simulink model "Fullcar_model_outdated"  (R2018b)
settings: Solver=FixedStepAuto  StartTime=0.0  StopTime=inf  FixedStep=0.002  RelTol=1e-3
PreLoadFcn:
  | fullcar_data
values from neighbouring files (symbols this model uses):
  Body_m = 1106.284    [fullcar_data.m]
  C_max = 4000    [fullcar_data.m]
  C_min = 300    [fullcar_data.m]
  N = L/B    [Fcn_General_Road.m]    (also in Road_Generator_Fullcar_final.m = floor(length(z_Rough_LH)/20); autoSaver.m = length(Road_z))
  s = (cnt - 1)*N    [Road_Generator_Fullcar_final.m]
  sat_limit = 1000    [fullcar_data.m]    (also in skyhook.m = 500)
  TW = 1568*0.001    (= 1.568)    [fullcar_data.m]
  WB = 2650*0.001    (= 2.65)    [fullcar_data.m]
  Whl_m_Frt = 101.488/2    (= 50.744)    [fullcar_data.m]
  Whl_m_Rr = 86.718/2    (= 43.359)    [fullcar_data.m]
  Y = zeros(N,4)    [autoSaver.m]
undefined symbols (not defined in the file or in its folder): X, Z
libraries: nesl_utility x43, sm_lib x36, sharedtransform x1
(part 2 of 2)

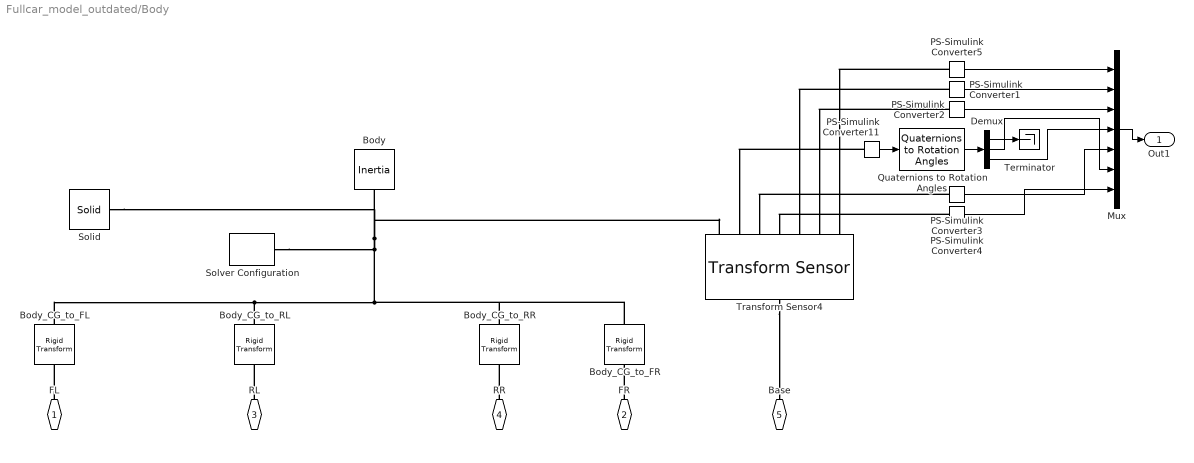
== system Fullcar_model_outdated/Body ==
  Body : sm_lib/Body Elements/Inertia  InertiaType=Custom  Mass=Body_m  MassUnits=kg  CenterOfMass=[0 0 0]  CenterOfMassUnits=m  MomentsOfInertia=[1 1 1]  MomentsOfInertiaUnits=kg*m^2  ProductsOfInertia=[0 0 0]  ProductsOfInertiaUnits=kg*m^2  GraphicType=Marker  MarkerShape=Inertia  MarkerSize=20  GraphicVisPropType=SimpleVisualProperties  GraphicDiffuseColor=[0.5 0.5 0.5]  GraphicSpecularColor=[0.5 0.5 0.5 1.0]  GraphicAmbientColor=[0.15 0.15 0.15 1.0]  GraphicEmissiveColor=[0.0 0.0 0.0 1.0]  GraphicShininess=75  GraphicOpacity=1.0
  Body_CG_to_FL : sm_lib/Frames and Transforms/Rigid Transform  TranslationMethod=Cartesian  TranslationStandardOffset=0  TranslationLengthUnit=m  TranslationStandardAxis=+Z  TranslationCartesianOffset=Body_CG_to_FL  TranslationROffset=0  TranslationROffsetUnits=m  TranslationZOffset=0  TranslationZOffsetUnits=m  TranslationThetaOffset=0  TranslationThetaOffsetUnits=deg  RotationMethod=None  RotationAngleUnits=deg  RotationStandardAxis=+Z  RotationAngle=0.0  RotationArbitraryAxis=[0 0 1]  FollAlignAxisA=+X  BaseAlignAxisA=+Y  FollAlignAxisB=+Y  BaseAlignAxisB=+Z  RotationSequenceAxes=FollowerAxes  RotationSequence=XYX  RotationSequenceAngles=[0 0 0]  RotationSequenceAnglesUnits=deg  RotationMatrix=[1 0 0; 0 1 0; 0 0 1]
  Body_CG_to_FR : sm_lib/Frames and Transforms/Rigid Transform  TranslationMethod=Cartesian  TranslationStandardOffset=0  TranslationLengthUnit=m  TranslationStandardAxis=+Z  TranslationCartesianOffset=Body_CG_to_FR  TranslationROffset=0  TranslationROffsetUnits=m  TranslationZOffset=0  TranslationZOffsetUnits=m  TranslationThetaOffset=0  TranslationThetaOffsetUnits=deg  RotationMethod=None  RotationAngleUnits=deg  RotationStandardAxis=+Z  RotationAngle=0.0  RotationArbitraryAxis=[0 0 1]  FollAlignAxisA=+X  BaseAlignAxisA=+Y  FollAlignAxisB=+Y  BaseAlignAxisB=+Z  RotationSequenceAxes=FollowerAxes  RotationSequence=XYX  RotationSequenceAngles=[0 0 0]  RotationSequenceAnglesUnits=deg  RotationMatrix=[1 0 0; 0 1 0; 0 0 1]
  Body_CG_to_RL : sm_lib/Frames and Transforms/Rigid Transform  TranslationMethod=Cartesian  TranslationStandardOffset=0  TranslationLengthUnit=m  TranslationStandardAxis=+Z  TranslationCartesianOffset=Body_CG_to_RL  TranslationROffset=0  TranslationROffsetUnits=m  TranslationZOffset=0  TranslationZOffsetUnits=m  TranslationThetaOffset=0  TranslationThetaOffsetUnits=deg  RotationMethod=None  RotationAngleUnits=deg  RotationStandardAxis=+Z  RotationAngle=0.0  RotationArbitraryAxis=[0 0 1]  FollAlignAxisA=+X  BaseAlignAxisA=+Y  FollAlignAxisB=+Y  BaseAlignAxisB=+Z  RotationSequenceAxes=FollowerAxes  RotationSequence=XYX  RotationSequenceAngles=[0 0 0]  RotationSequenceAnglesUnits=deg  RotationMatrix=[1 0 0; 0 1 0; 0 0 1]
  Body_CG_to_RR : sm_lib/Frames and Transforms/Rigid Transform  TranslationMethod=Cartesian  TranslationStandardOffset=0  TranslationLengthUnit=m  TranslationStandardAxis=+Z  TranslationCartesianOffset=Body_CG_to_RR  TranslationROffset=0  TranslationROffsetUnits=m  TranslationZOffset=0  TranslationZOffsetUnits=m  TranslationThetaOffset=0  TranslationThetaOffsetUnits=deg  RotationMethod=None  RotationAngleUnits=deg  RotationStandardAxis=+Z  RotationAngle=0.0  RotationArbitraryAxis=[0 0 1]  FollAlignAxisA=+X  BaseAlignAxisA=+Y  FollAlignAxisB=+Y  BaseAlignAxisB=+Z  RotationSequenceAxes=FollowerAxes  RotationSequence=XYX  RotationSequenceAngles=[0 0 0]  RotationSequenceAnglesUnits=deg  RotationMatrix=[1 0 0; 0 1 0; 0 0 1]
  Demux : Demux  Outputs=3
  Mux : Mux  Inputs=7
  PS-Simulink Converter{1..5,11} (6 alike) : nesl_utility/PS-Simulink Converter  PhysicalDomain=network_engine_domain  SubClassName=ps_output  LeftPortType=input  RightPortType=output  PseudoPeriodic=off  Frequencies=[]  Unit=1  AffineConversion=off
  Quaternions to Rotation Angles : sharedtransform/Quaternions to Rotation Angles  rotationOrder=ZYX  aMode=aMode
      settings: SourceProductBaseCode=AE
  Solid : sm_lib/Body Elements/Solid  InertiaType=CalculateFromGeometry  Mass=1  MassUnits=kg  CenterOfMass=[0 0 0]  CenterOfMassUnits=m  MomentsOfInertia=[1 1 1]  MomentsOfInertiaUnits=kg*m^2  ProductsOfInertia=[0 0 0]  ProductsOfInertiaUnits=kg*m^2  BasedOnType=Density  Density=1000  DensityUnits=kg/m^3  DoExposeReferenceFrame=on  SerializedFrames=<Frames/>  GraphicType=FromGeometry  MarkerShape=Sphere  MarkerSize=10  GraphicVisPropType=SimpleVisualProperties  GraphicDiffuseColor=[0.8 1.0 0.8]  GraphicSpecularColor=[0.5 0.5 0.5 1.0]  GraphicAmbientColor=[0.15 0.15 0.15 1.0]  GraphicEmissiveColor=[0.0 0.0 0.0 1.0]  GraphicShininess=75  GraphicOpacity=0.5  GeometryShape=Brick  RectangleSize=[1 1]  RectangleSizeUnits=m  BrickDimensions=[WB TW 0.5]  BrickDimensionUnits=m  CylinderRadius=1  CylinderRadiusUnits=m  CylinderLength=1  CylinderLengthUnits=m  SphereRadius=1  SphereRadiusUnits=m  EllipsoidRadii=[1 1 1]  EllipsoidRadiiUnits=m  ExtrusionCrossSection=[1 1; -1 1; -1 -1; 1 -1]  ExtrusionCrossSectionUnits=m  ExtrusionLength=1  ExtrusionLengthUnits=m  PolygonNumSides=3  PolygonOuterRadius=1  PolygonOuterRadiusUnits=m  ExtGeomFileType=STEP  ExtGeomFileUnits=m  RevolutionCrossSection=[1 1; 1 -1; 2 -1; 2 1]  RevolutionCrossSectionUnits=m  RevolutionExtent=Full  RevolutionAngle=180  RevolutionAngleUnits=deg
  Solver Configuration : nesl_utility/Solver Configuration  PhysicalDomain=network_engine_domain  SubClassName=solver  LeftPortType=input  RightPortType=generic  Tones=[]  Harmonics=[]  SimulateNoise=off  Profile=off  UseLocalSampling=off  EnableSwitchedLinearOptims=on  FrequencyDomain=off  UseCCode=off  RelTol=0.001  AbsTol=1e-06  MinStep=1e-09  ToWorkspace=off  RevertToSquareIcSolve=off  NumHomotopyIterations=100  PhasorMode=off  PhasorModeNumHarmonics=1  DoDC=off  ResidualTolerance=1e-09  UseLocalSolver=off  LocalSolverChoice=NE_BACKWARD_EULER_ADVANCER  LocalSolverSampleTime=0.001  DoFixedCost=off  MaxNonlinIter=3  MaxModeIter=2  LinearAlgebra=auto  EquationFormulation=NE_TIME_EF  DelaysMemoryBudget=1024  AutomaticFiltering=on  FilteringTimeConstant=0.001  PartitionStorageMethod=AS_NEEDED  PartitionMemoryBudget=1024  PartitionMethod=FAST
  Terminator : Terminator
  Transform Sensor4 : sm_lib/Frames and Transforms/Transform Sensor  MeasurementFrame=World  SenseAngle=off  SenseAxis=off  SenseAngle1=off  SenseAngle2=off  SenseAngle3=off  SenseQ=on  SenseR=off  SenseOmegaX=on  SenseOmegaY=on  SenseOmegaZ=off  SenseOmega1=off  SenseOmega2=off  SenseOmega3=off  SenseQDot=off  SenseRDot=off  SenseAlphaX=off  SenseAlphaY=off  SenseAlphaZ=off  SenseAlpha1=off  SenseAlpha2=off  SenseAlpha3=off  SenseQDDot=off  SenseRDDot=off  SenseX=off  SenseY=off  SenseZ=on  SenseRad=off  SenseAzim=off  SenseDist=off  SenseInc=off  SenseXDot=off  SenseYDot=off  SenseZDot=on  SenseRadDot=off  SenseAzimDot=off  SenseDistDot=off  SenseIncDot=off  SenseXDDot=off  SenseYDDot=off  SenseZDDot=on  SenseRadDDot=off  SenseAzimDDot=off  SenseDistDDot=off  SenseIncDDot=off
  FL : PMIOPort  Side=Left
  FR : PMIOPort  Port=2  Side=Right
  RL : PMIOPort  Port=3  Side=Left
  RR : PMIOPort  Port=4  Side=Right
  Base : PMIOPort  Port=5  Side=Right
  Out1 : Outport
  wires:
  Demux/3 -> Mux/4
  PS-Simulink Converter11/1 -> Quaternions to Rotation Angles/1
  Quaternions to Rotation Angles/1 -> Demux/1
  Demux/1 -> Terminator/1
  PS-Simulink Converter2/1 -> Mux/3
  PS-Simulink Converter3/1 -> Mux/5
  Mux/1 -> Out1/1
  Demux/2 -> Mux/6
  PS-Simulink Converter1/1 -> Mux/2
  PS-Simulink Converter4/1 -> Mux/7
  PS-Simulink Converter5/1 -> Mux/1
  connections:
  Body_CG_to_FL/LConn1 -- Body_CG_to_RL/LConn1 -- Body_CG_to_RR/LConn1 -- Body_CG_to_FR/LConn1 -- Body/RConn1 -- Solid/RConn1 -- Transform Sensor4/RConn1 -- Solver Configuration/RConn1
  FR/RConn1 -- Body_CG_to_FR/RConn1
  FL/RConn1 -- Body_CG_to_FL/RConn1
  RL/RConn1 -- Body_CG_to_RL/RConn1
  RR/RConn1 -- Body_CG_to_RR/RConn1
  PS-Simulink Converter1/LConn1 -- Transform Sensor4/RConn5
  PS-Simulink Converter3/LConn1 -- Transform Sensor4/RConn3
  PS-Simulink Converter4/LConn1 -- Transform Sensor4/RConn4
  PS-Simulink Converter2/LConn1 -- Transform Sensor4/RConn6
  PS-Simulink Converter11/LConn1 -- Transform Sensor4/RConn2
  Transform Sensor4/LConn1 -- Base/RConn1
  PS-Simulink Converter5/LConn1 -- Transform Sensor4/RConn7

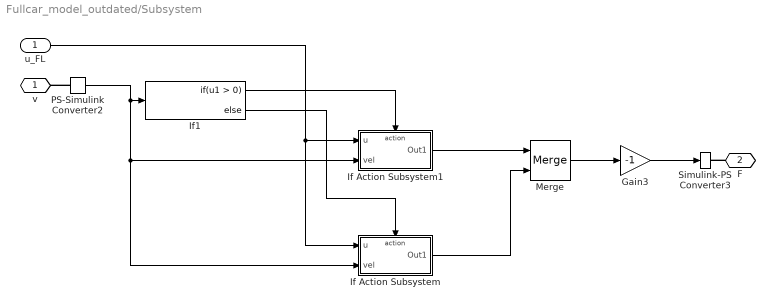
== system Fullcar_model_outdated/Subsystem ==
  "u_FL " : Inport
  Gain3 : Gain  Gain=-1
  If Action Subsystem : Subsystem  TreatAsAtomicUnit=on
  If Action Subsystem1 : Subsystem  TreatAsAtomicUnit=on
  If1 : If
  Merge : Merge
  PS-Simulink Converter2 : nesl_utility/PS-Simulink Converter  PhysicalDomain=network_engine_domain  SubClassName=ps_output  LeftPortType=input  RightPortType=output  PseudoPeriodic=off  Frequencies=[]  Unit=1  AffineConversion=off
  Simulink-PS Converter3 : nesl_utility/Simulink-PS Converter  PhysicalDomain=network_engine_domain  SubClassName=ps_input  LeftPortType=input  RightPortType=output  PseudoPeriodic=off  Frequencies=[]  NoiseDistribution=none  NoiseParameters=[]  Unit=1  AffineConversion=off  FilteringAndDerivatives=provide  SimscapeFilterOrder=1  InputFilterTimeConstant=0.001  UdotUserProvided=0
  "v " : PMIOPort  Side=Left
  F : PMIOPort  Port=2  Side=Right
  wires:
  PS-Simulink Converter2/1 -> If Action Subsystem/2("vel "), If Action Subsystem1/2("vel "), If1/1
  If1/1 -> If Action Subsystem1/Action
  Merge/1 -> Gain3/1
  If Action Subsystem1/1(Out1) -> Merge/1
  If1/2 -> If Action Subsystem/Action
  "u_FL "/1 -> If Action Subsystem/1("u "), If Action Subsystem1/1("u ")
  If Action Subsystem/1(Out1) -> Merge/2
  Gain3/1 -> Simulink-PS Converter3/1
  connections:
  PS-Simulink Converter2/LConn1 -- "v "/RConn1
  F/RConn1 -- Simulink-PS Converter3/RConn1

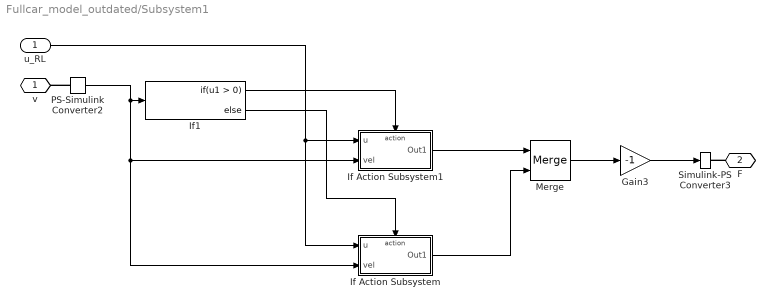
== system Fullcar_model_outdated/Subsystem1 ==
  "u_RL " : Inport
  Gain3 : Gain  Gain=-1
  If Action Subsystem : Subsystem  TreatAsAtomicUnit=on
  If Action Subsystem1 : Subsystem  TreatAsAtomicUnit=on
  If1 : If
  Merge : Merge
  PS-Simulink Converter2 : nesl_utility/PS-Simulink Converter  PhysicalDomain=network_engine_domain  SubClassName=ps_output  LeftPortType=input  RightPortType=output  PseudoPeriodic=off  Frequencies=[]  Unit=1  AffineConversion=off
  Simulink-PS Converter3 : nesl_utility/Simulink-PS Converter  PhysicalDomain=network_engine_domain  SubClassName=ps_input  LeftPortType=input  RightPortType=output  PseudoPeriodic=off  Frequencies=[]  NoiseDistribution=none  NoiseParameters=[]  Unit=1  AffineConversion=off  FilteringAndDerivatives=provide  SimscapeFilterOrder=1  InputFilterTimeConstant=0.001  UdotUserProvided=0
  "v " : PMIOPort  Side=Left
  F : PMIOPort  Port=2  Side=Right
  wires:
  PS-Simulink Converter2/1 -> If Action Subsystem/2("vel "), If Action Subsystem1/2("vel "), If1/1
  If1/1 -> If Action Subsystem1/Action
  Merge/1 -> Gain3/1
  If Action Subsystem1/1(Out1) -> Merge/1
  If1/2 -> If Action Subsystem/Action
  "u_RL "/1 -> If Action Subsystem/1("u "), If Action Subsystem1/1("u ")
  If Action Subsystem/1(Out1) -> Merge/2
  Gain3/1 -> Simulink-PS Converter3/1
  connections:
  PS-Simulink Converter2/LConn1 -- "v "/RConn1
  F/RConn1 -- Simulink-PS Converter3/RConn1

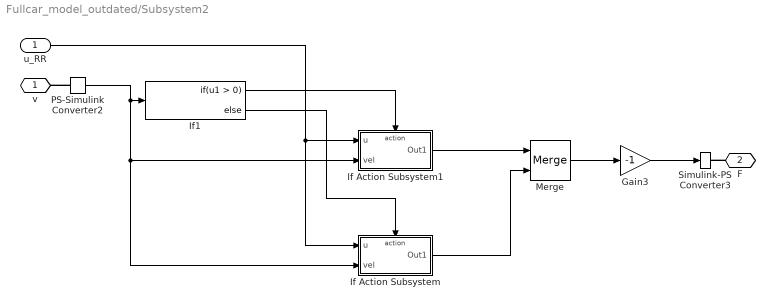
== system Fullcar_model_outdated/Subsystem2 ==
  "u_RR " : Inport
  Gain3 : Gain  Gain=-1
  If Action Subsystem : Subsystem  TreatAsAtomicUnit=on
  If Action Subsystem1 : Subsystem  TreatAsAtomicUnit=on
  If1 : If
  Merge : Merge
  PS-Simulink Converter2 : nesl_utility/PS-Simulink Converter  PhysicalDomain=network_engine_domain  SubClassName=ps_output  LeftPortType=input  RightPortType=output  PseudoPeriodic=off  Frequencies=[]  Unit=1  AffineConversion=off
  Simulink-PS Converter3 : nesl_utility/Simulink-PS Converter  PhysicalDomain=network_engine_domain  SubClassName=ps_input  LeftPortType=input  RightPortType=output  PseudoPeriodic=off  Frequencies=[]  NoiseDistribution=none  NoiseParameters=[]  Unit=1  AffineConversion=off  FilteringAndDerivatives=provide  SimscapeFilterOrder=1  InputFilterTimeConstant=0.001  UdotUserProvided=0
  "v " : PMIOPort  Side=Left
  F : PMIOPort  Port=2  Side=Right
  wires:
  PS-Simulink Converter2/1 -> If Action Subsystem/2("vel "), If Action Subsystem1/2("vel "), If1/1
  If1/1 -> If Action Subsystem1/Action
  Merge/1 -> Gain3/1
  If Action Subsystem1/1(Out1) -> Merge/1
  If1/2 -> If Action Subsystem/Action
  "u_RR "/1 -> If Action Subsystem/1("u "), If Action Subsystem1/1("u ")
  If Action Subsystem/1(Out1) -> Merge/2
  Gain3/1 -> Simulink-PS Converter3/1
  connections:
  PS-Simulink Converter2/LConn1 -- "v "/RConn1
  F/RConn1 -- Simulink-PS Converter3/RConn1

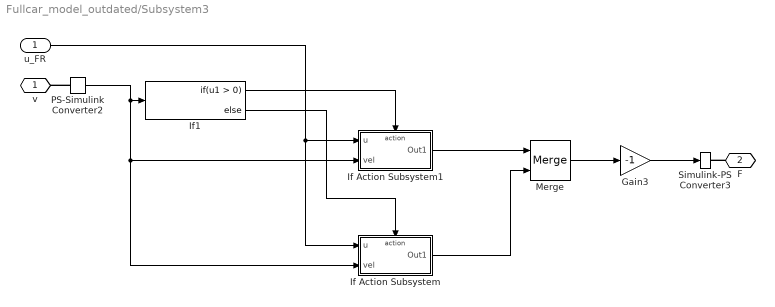
== system Fullcar_model_outdated/Subsystem3 ==
  "u_FR " : Inport
  Gain3 : Gain  Gain=-1
  If Action Subsystem : Subsystem  TreatAsAtomicUnit=on
  If Action Subsystem1 : Subsystem  TreatAsAtomicUnit=on
  If1 : If
  Merge : Merge
  PS-Simulink Converter2 : nesl_utility/PS-Simulink Converter  PhysicalDomain=network_engine_domain  SubClassName=ps_output  LeftPortType=input  RightPortType=output  PseudoPeriodic=off  Frequencies=[]  Unit=1  AffineConversion=off
  Simulink-PS Converter3 : nesl_utility/Simulink-PS Converter  PhysicalDomain=network_engine_domain  SubClassName=ps_input  LeftPortType=input  RightPortType=output  PseudoPeriodic=off  Frequencies=[]  NoiseDistribution=none  NoiseParameters=[]  Unit=1  AffineConversion=off  FilteringAndDerivatives=provide  SimscapeFilterOrder=1  InputFilterTimeConstant=0.001  UdotUserProvided=0
  "v " : PMIOPort  Side=Left
  F : PMIOPort  Port=2  Side=Right
  wires:
  PS-Simulink Converter2/1 -> If Action Subsystem/2("vel "), If Action Subsystem1/2("vel "), If1/1
  If1/1 -> If Action Subsystem1/Action
  Merge/1 -> Gain3/1
  If Action Subsystem1/1(Out1) -> Merge/1
  If1/2 -> If Action Subsystem/Action
  "u_FR "/1 -> If Action Subsystem/1("u "), If Action Subsystem1/1("u ")
  If Action Subsystem/1(Out1) -> Merge/2
  Gain3/1 -> Simulink-PS Converter3/1
  connections:
  PS-Simulink Converter2/LConn1 -- "v "/RConn1
  F/RConn1 -- Simulink-PS Converter3/RConn1

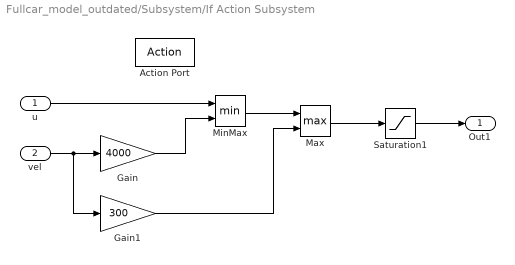
== system Fullcar_model_outdated/Subsystem/If Action Subsystem ==
  "u " : Inport
  "vel " : Inport  Port=2
  Action Port : ActionPort
  Gain : Gain  Gain=4000
  Gain1 : Gain  Gain=300
  Max : MinMax  Function=max  Inputs=2
  MinMax : MinMax  Inputs=2
  Saturation1 : Saturate  UpperLimit=sat_limit  LowerLimit=-sat_limit
  Out1 : Outport
  wires:
  Gain/1 -> MinMax/2
  Gain1/1 -> Max/2
  "vel "/1 -> Gain1/1, Gain/1
  "u "/1 -> MinMax/1
  Max/1 -> Saturation1/1
  MinMax/1 -> Max/1
  Saturation1/1 -> Out1/1

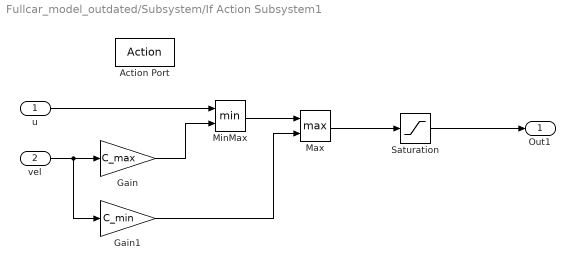
== system Fullcar_model_outdated/Subsystem/If Action Subsystem1 ==
  "u " : Inport
  "vel " : Inport  Port=2
  Action Port : ActionPort
  Gain : Gain  Gain=C_max
  Gain1 : Gain  Gain=C_min
  Max : MinMax  Function=max  Inputs=2
  MinMax : MinMax  Inputs=2
  Saturation : Saturate  UpperLimit=sat_limit  LowerLimit=-sat_limit
  Out1 : Outport
  wires:
  "u "/1 -> MinMax/1
  MinMax/1 -> Max/1
  Max/1 -> Saturation/1
  "vel "/1 -> Gain1/1, Gain/1
  Gain/1 -> MinMax/2
  Gain1/1 -> Max/2
  Saturation/1 -> Out1/1

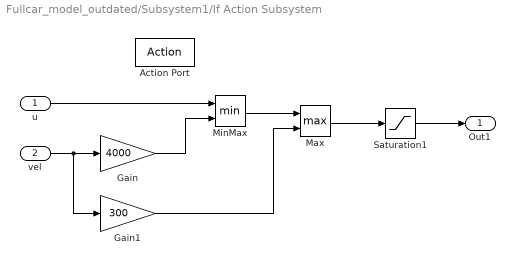
== system Fullcar_model_outdated/Subsystem1/If Action Subsystem ==
  "u " : Inport
  "vel " : Inport  Port=2
  Action Port : ActionPort
  Gain : Gain  Gain=4000
  Gain1 : Gain  Gain=300
  Max : MinMax  Function=max  Inputs=2
  MinMax : MinMax  Inputs=2
  Saturation1 : Saturate  UpperLimit=sat_limit  LowerLimit=-sat_limit
  Out1 : Outport
  wires:
  Gain/1 -> MinMax/2
  Gain1/1 -> Max/2
  "vel "/1 -> Gain1/1, Gain/1
  "u "/1 -> MinMax/1
  Max/1 -> Saturation1/1
  MinMax/1 -> Max/1
  Saturation1/1 -> Out1/1

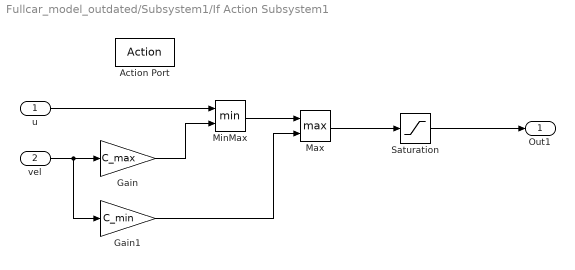
== system Fullcar_model_outdated/Subsystem1/If Action Subsystem1 ==
  "u " : Inport
  "vel " : Inport  Port=2
  Action Port : ActionPort
  Gain : Gain  Gain=C_max
  Gain1 : Gain  Gain=C_min
  Max : MinMax  Function=max  Inputs=2
  MinMax : MinMax  Inputs=2
  Saturation : Saturate  UpperLimit=sat_limit  LowerLimit=-sat_limit
  Out1 : Outport
  wires:
  "u "/1 -> MinMax/1
  MinMax/1 -> Max/1
  Max/1 -> Saturation/1
  "vel "/1 -> Gain1/1, Gain/1
  Gain/1 -> MinMax/2
  Gain1/1 -> Max/2
  Saturation/1 -> Out1/1

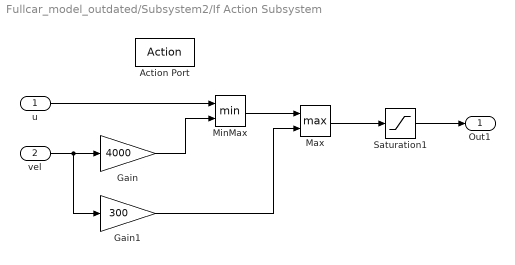
== system Fullcar_model_outdated/Subsystem2/If Action Subsystem ==
  "u " : Inport
  "vel " : Inport  Port=2
  Action Port : ActionPort
  Gain : Gain  Gain=4000
  Gain1 : Gain  Gain=300
  Max : MinMax  Function=max  Inputs=2
  MinMax : MinMax  Inputs=2
  Saturation1 : Saturate  UpperLimit=sat_limit  LowerLimit=-sat_limit
  Out1 : Outport
  wires:
  Gain/1 -> MinMax/2
  Gain1/1 -> Max/2
  "vel "/1 -> Gain1/1, Gain/1
  "u "/1 -> MinMax/1
  Max/1 -> Saturation1/1
  MinMax/1 -> Max/1
  Saturation1/1 -> Out1/1

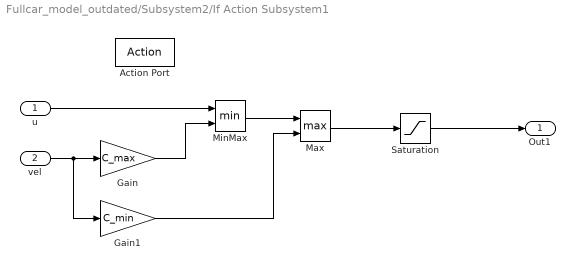
== system Fullcar_model_outdated/Subsystem2/If Action Subsystem1 ==
  "u " : Inport
  "vel " : Inport  Port=2
  Action Port : ActionPort
  Gain : Gain  Gain=C_max
  Gain1 : Gain  Gain=C_min
  Max : MinMax  Function=max  Inputs=2
  MinMax : MinMax  Inputs=2
  Saturation : Saturate  UpperLimit=sat_limit  LowerLimit=-sat_limit
  Out1 : Outport
  wires:
  "u "/1 -> MinMax/1
  MinMax/1 -> Max/1
  Max/1 -> Saturation/1
  "vel "/1 -> Gain1/1, Gain/1
  Gain/1 -> MinMax/2
  Gain1/1 -> Max/2
  Saturation/1 -> Out1/1

== system Fullcar_model_outdated/Subsystem3/If Action Subsystem ==
  "u " : Inport
  "vel " : Inport  Port=2
  Action Port : ActionPort
  Gain : Gain  Gain=4000
  Gain1 : Gain  Gain=300
  Max : MinMax  Function=max  Inputs=2
  MinMax : MinMax  Inputs=2
  Saturation1 : Saturate  UpperLimit=sat_limit  LowerLimit=-sat_limit
  Out1 : Outport
  wires:
  Gain/1 -> MinMax/2
  Gain1/1 -> Max/2
  "vel "/1 -> Gain1/1, Gain/1
  "u "/1 -> MinMax/1
  Max/1 -> Saturation1/1
  MinMax/1 -> Max/1
  Saturation1/1 -> Out1/1

== system Fullcar_model_outdated/Subsystem3/If Action Subsystem1 ==
  "u " : Inport
  "vel " : Inport  Port=2
  Action Port : ActionPort
  Gain : Gain  Gain=C_max
  Gain1 : Gain  Gain=C_min
  Max : MinMax  Function=max  Inputs=2
  MinMax : MinMax  Inputs=2
  Saturation : Saturate  UpperLimit=sat_limit  LowerLimit=-sat_limit
  Out1 : Outport
  wires:
  "u "/1 -> MinMax/1
  MinMax/1 -> Max/1
  Max/1 -> Saturation/1
  "vel "/1 -> Gain1/1, Gain/1
  Gain/1 -> MinMax/2
  Gain1/1 -> Max/2
  Saturation/1 -> Out1/1
